simulink model "SamplePartsB"  (R2023a)
settings: configuration reference "TrStd_common_Mil_confset" (kept outside this file)
settings Model: DataDictionary=Sample_common_config.sldd  Creator=C9166  LastModifiedBy=C9166
settings ConfigSetRef: SourceName=TrStd_common_Mil_confset

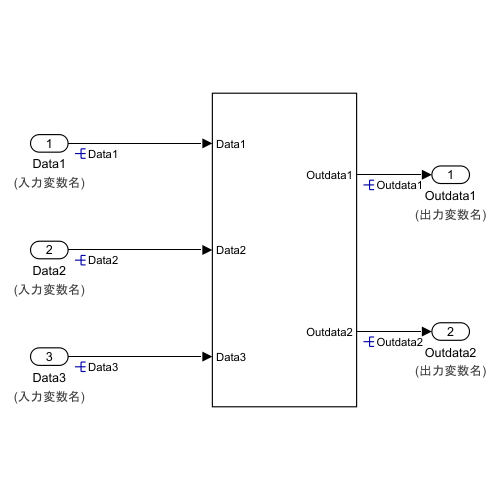
[thumbnail: Simulink's stored preview of the top-level diagram]
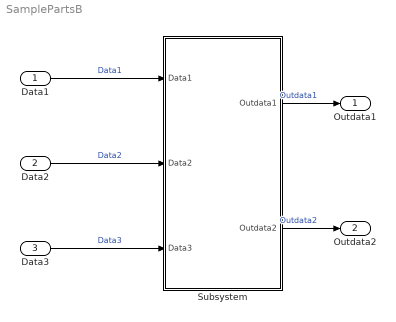
== system SamplePartsB ==
  Data1 : Inport  Description=入力変数名
      settings: AttributesFormatString=(%<Description>)
  Data2 : Inport  Description=入力変数名  Port=2
      settings: AttributesFormatString=(%<Description>)
  Data3 : Inport  Description=入力変数名  Port=3
      settings: AttributesFormatString=(%<Description>)
  Subsystem : Subsystem
  Outdata1 : Outport  Description=出力変数名
      settings: AttributesFormatString=(%<Description>)
  Outdata2 : Outport  Description=出力変数名  Port=2
      settings: AttributesFormatString=(%<Description>)
  wires:
  Data1/1 -> Subsystem/1(Data1)  "Data1"
  Data2/1 -> Subsystem/2(Data2)  "Data2"
  Data3/1 -> Subsystem/3(Data3)  "Data3"
  Subsystem/1(Outdata1) -> Outdata1/1  "Outdata1"
  Subsystem/2(Outdata2) -> Outdata2/1  "Outdata2"

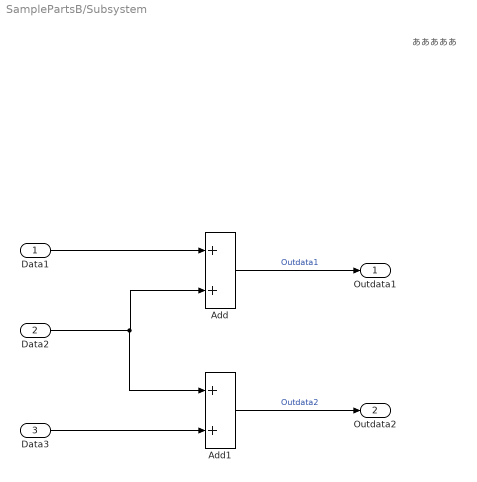
== system SamplePartsB/Subsystem ==
  note: あああああ
  Data1 : Inport
  Data2 : Inport  Port=2
  Data3 : Inport  Port=3
  Add : Sum  InputSameDT=on  RndMeth=Simplest
  Add1 : Sum  InputSameDT=on  RndMeth=Simplest
  Outdata1 : Outport
  Outdata2 : Outport  Port=2
  wires:
  Data3/1 -> Add1/2
  Data2/1 -> Add1/1, Add/2
  Data1/1 -> Add/1
  Add1/1 -> Outdata2/1  "Outdata2"
  Add/1 -> Outdata1/1  "Outdata1"
